simulink model "thrustandflapping_model"  (Simulink 7.7)
settings: Solver=ode45  StartTime=0.0  StopTime=12  RelTol=1e-3
settings Model: Creator=Administrator  LastModifiedBy=Administrator

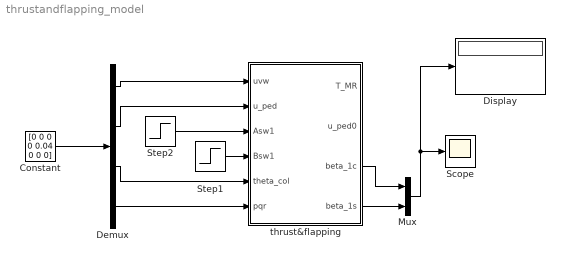
== system thrustandflapping_model ==
  Constant : Constant  Value=[0 0 0 0 0.04 0 0 0]
  Demux : Demux  Outputs=[3 1 1 3]
  Display : Display
  Mux : Mux  Inputs=2
  Scope : Scope
      settings: YMin=-0.8  YMax=0.9
  Step1 : Step  Time=0.5  SampleTime=0
  Step2 : Step  Time=0.5  SampleTime=0
  thrust&flapping : Subsystem  mask{Ksw=0.2, Kcr=0.8, T_old=50, vi0=10}
  wires:
  Constant/1 -> Demux/1
  Demux/1 -> thrust&flapping/1(uvw)
  Demux/2 -> thrust&flapping/2(u_ped)
  Demux/3 -> thrust&flapping/5(theta_col)
  Demux/4 -> thrust&flapping/6(pqr)
  Step2/1 -> thrust&flapping/3(Asw1)
  Step1/1 -> thrust&flapping/4(Bsw1)
  thrust&flapping/3(beta_1c) -> Mux/1
  thrust&flapping/4(beta_1s) -> Mux/2
  Mux/1 -> Scope/1, Display/1

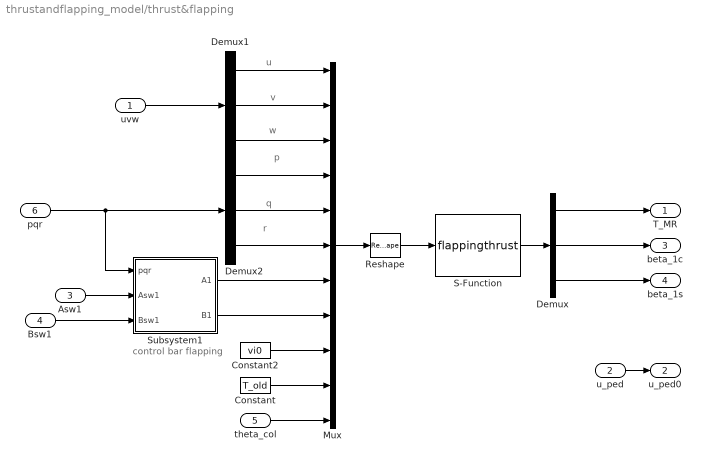
== system thrustandflapping_model/thrust&flapping ==
  note: p
  note: q
  note: r
  note: u
  note: v
  note: w
  note: control bar flapping
  uvw : Inport
  u_ped : Inport  Port=2
  Asw1 : Inport  Port=3
  Bsw1 : Inport  Port=4
  theta_col : Inport  Port=5
  pqr : Inport  Port=6
  Constant : Constant  Value=T_old
  Constant2 : Constant  Value=vi0
  Demux : Demux  Outputs=3
  Demux1 : Demux  Outputs=[1 1 1 ]
  Demux2 : Demux  Outputs=[1 1 1 ]
  Mux : Mux  Inputs=11
  Reshape : Reshape  OutputDimensionality=Column vector (2-D)
  S-Function : S-Function  RequirementInfo={} %GIDa_ecab073c_cbac_40c6_823c_865874bfc3b3  FunctionName=flappingthrust  EnableBusSupport=off
  Subsystem1 : Subsystem
  T_MR : Outport
  u_ped0 : Outport  Port=2
  beta_1c : Outport  Port=3
  beta_1s : Outport  Port=4
  wires:
  u_ped/1 -> u_ped0/1
  S-Function/1 -> Demux/1
  Demux/1 -> T_MR/1
  Demux/2 -> beta_1c/1
  Demux1/1 -> Mux/1
  Demux1/2 -> Mux/2
  Demux1/3 -> Mux/3
  uvw/1 -> Demux1/1
  Demux2/1 -> Mux/4
  Demux2/2 -> Mux/5
  Demux2/3 -> Mux/6
  pqr/1 -> Demux2/1, Subsystem1/1(pqr)
  Constant2/1 -> Mux/9
  theta_col/1 -> Mux/11
  Demux/3 -> beta_1s/1
  Constant/1 -> Mux/10
  Mux/1 -> Reshape/1
  Reshape/1 -> S-Function/1
  Subsystem1/1(A1) -> Mux/7
  Subsystem1/2(B1) -> Mux/8
  Asw1/1 -> Subsystem1/2(Asw1)
  Bsw1/1 -> Subsystem1/3(Bsw1)

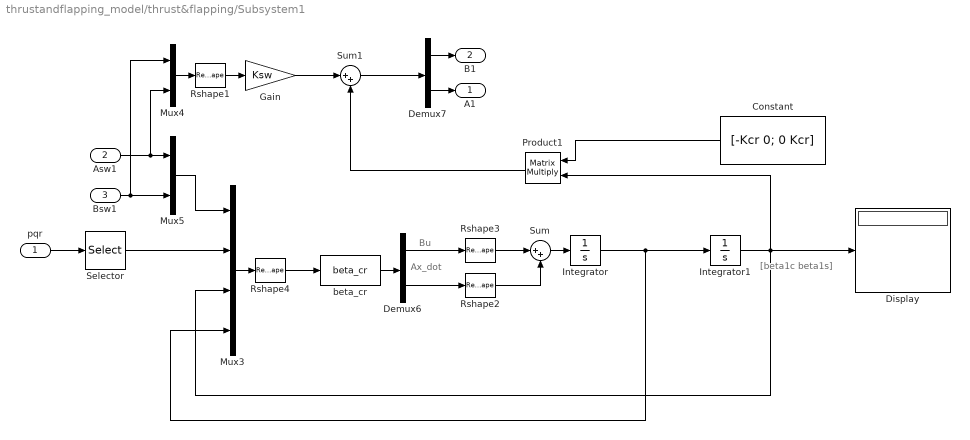
== system thrustandflapping_model/thrust&flapping/Subsystem1 ==
  note: Ax_dot
  note: Bu
  note: [beta1c
      | beta1s]
  pqr : Inport
  Asw1 : Inport  Port=2
  Bsw1 : Inport  Port=3
  Constant : Constant  Value=[-Kcr 0; 0 Kcr]
  Demux6 : Demux  Outputs=[2 2]
  Demux7 : Demux  Outputs=[1 1]
  Display : Display
  Gain : Gain  Gain=Ksw
  Integrator : Integrator  InitialCondition=[0;0]
  Integrator1 : Integrator  InitialCondition=[0;0]
  Mux3 : Mux
  Mux4 : Mux  Inputs=2
  Mux5 : Mux  Inputs=2
  Product1 : Product  Multiplication=Matrix(*)  RndMeth=Zero
  Rshape{1..4} (4 alike) : Reshape  OutputDimensionality=Column vector (2-D)
  Selector : Selector  InputPortWidth=3  IndexOptions=Index vector (dialog)  Indices=[1 2]  OutputSizes=1
  Sum : Sum  Inputs=|++
  Sum1 : Sum  Inputs=|++
  beta_cr : S-Function  FunctionName=beta_cr  EnableBusSupport=off
  A1 : Outport
  B1 : Outport  Port=2
  wires:
  Rshape4/1 -> beta_cr/1
  Mux3/1 -> Rshape4/1
  Rshape2/1 -> Sum/2
  Rshape3/1 -> Sum/1
  Demux6/2 -> Rshape2/1
  Demux6/1 -> Rshape3/1
  Selector/1 -> Mux3/2
  Mux5/1 -> Mux3/1
  pqr/1 -> Selector/1
  Demux7/2 -> A1/1
  Demux7/1 -> B1/1
  Product1/1 -> Sum1/2
  Mux4/1 -> Rshape1/1
  Rshape1/1 -> Gain/1
  Sum1/1 -> Demux7/1
  Gain/1 -> Sum1/1
  Constant/1 -> Product1/1
  Sum/1 -> Integrator/1
  beta_cr/1 -> Demux6/1
  Integrator1/1 -> Product1/2, Mux3/3, Display/1
  Integrator/1 -> Mux3/4, Integrator1/1
  Bsw1/1 -> Mux5/2, Mux4/1
  Asw1/1 -> Mux5/1, Mux4/2
